simulink model "problem2Simulink"  (R2022a)
settings: Solver=VariableStepAuto  StartTime=0.0  StopTime=10.0  FixedStep=0.001  RelTol=1e-3
settings Model: Creator=ianmf  LastModifiedBy=ianmf

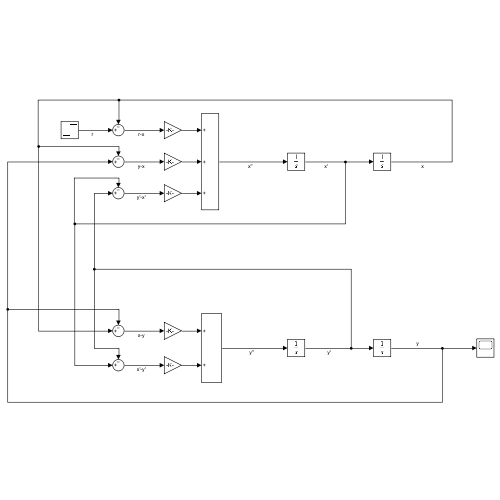
[thumbnail: Simulink's stored preview of the top-level diagram]
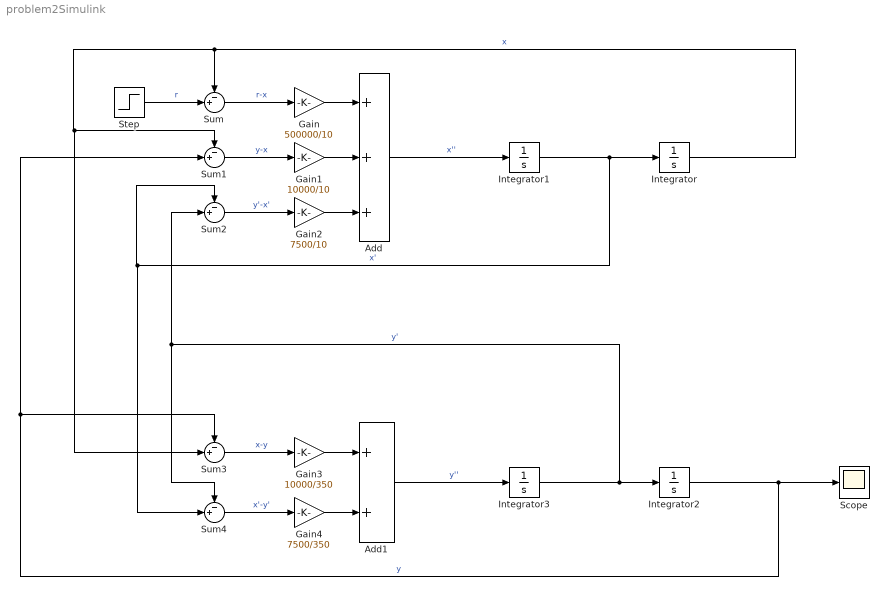
== system problem2Simulink ==
  Add : Sum  Inputs=+++
  Add1 : Sum
  Gain : Gain  Gain=500000/10
  Gain1 : Gain  Gain=10000/10
  Gain2 : Gain  Gain=7500/10
  Gain3 : Gain  Gain=10000/350
  Gain4 : Gain  Gain=7500/350
  Integrator{,1..3} (4 alike) : Integrator
  Scope : Scope
  Step : Step  Time=5  SampleTime=0
  Sum{,1..4} (5 alike) : Sum  Inputs=-+|
  wires:
  Integrator1/1 -> Sum4/2, Sum2/1, Integrator/1  "x'"
  Integrator3/1 -> Sum4/1, Sum2/2, Integrator2/1  "y'"
  Add/1 -> Integrator1/1  "x''"
  Gain2/1 -> Add/3
  Gain1/1 -> Add/2
  Gain/1 -> Add/1
  Step/1 -> Sum/2  "r"
  Sum/1 -> Gain/1  "r-x"
  Integrator/1 -> Sum/1, Sum3/2, Sum1/1  "x"
  Sum1/1 -> Gain1/1  "y-x"
  Sum2/1 -> Gain2/1  "y'-x'"
  Add1/1 -> Integrator3/1  "y''"
  Gain3/1 -> Add1/1
  Gain4/1 -> Add1/2
  Sum3/1 -> Gain3/1  "x-y"
  Sum4/1 -> Gain4/1  "x'-y'"
  Integrator2/1 -> Sum3/1, Sum1/2, Scope/1  "y"
